simulink model "lab4_part1_question3"  (R2023a)
settings: Solver=VariableStepAuto  StartTime=0.0  StopTime=0.1  RelTol=1e-3
libraries: dspfdesign x1
settings Model: Creator=ma_kaba  LastModifiedBy=ma_kaba

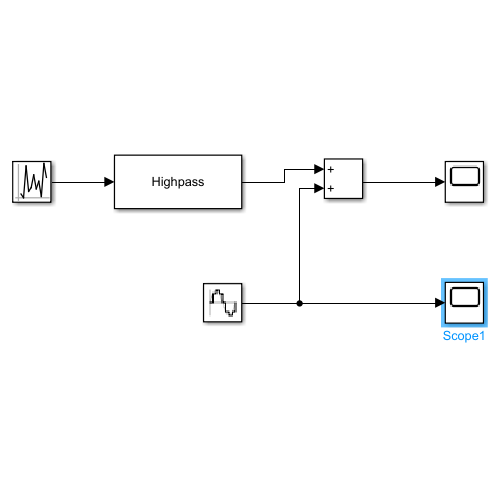
[thumbnail: Simulink's stored preview of the top-level diagram]
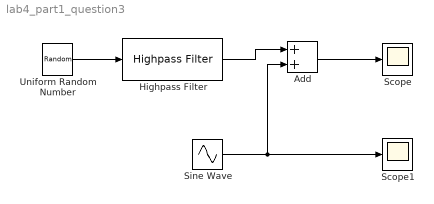
== system lab4_part1_question3 ==
  Add : Sum
  Highpass Filter : dspfdesign/Highpass Filter  FilterType=IIR  DesignForMinimumOrder=on  FilterOrder=50  StopbandFrequency=3600  PassbandFrequency=3800  StopbandAttenuation=60  PassbandRipple=1  SampleRateMode=Specify on dialog  SampleRate=8000  SimulateUsing=Interpreted execution  roundingMode=Floor  coeffsDataTypeStr=fixdt(1,16)
  Scope : Scope
  Scope1 : Scope
  Sine Wave : Sin  Frequency=2*pi*100  SampleTime=1/8000
  Uniform Random Number : UniformRandomNumber  Minimum=-5  Maximum=5  SampleTime=1/8000
  wires:
  Uniform Random Number/1 -> Highpass Filter/1
  Sine Wave/1 -> Scope1/1, Add/2
  Highpass Filter/1 -> Add/1
  Add/1 -> Scope/1
